simulink model "bai2111"  (R2022b)
settings: Solver=VariableStepAuto  StartTime=0.0  StopTime=20  RelTol=1e-8
values from neighbouring files (symbols this model uses):
  k0 = -8    [bai21111.m]
  k1 = -1    [bai21111.m]
  T = T_list(k)    [bai21111.m]
settings Model: Creator=admin  LastModifiedBy=admin

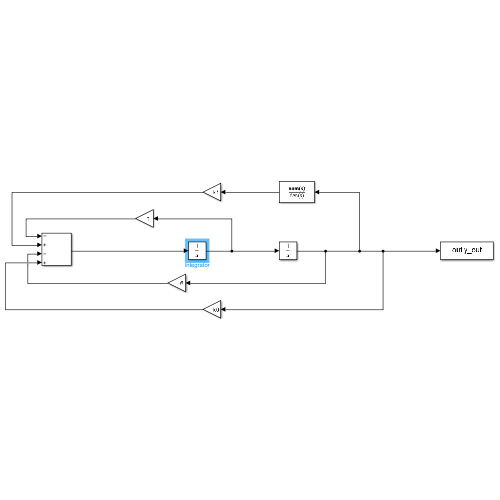
[thumbnail: Simulink's stored preview of the top-level diagram]
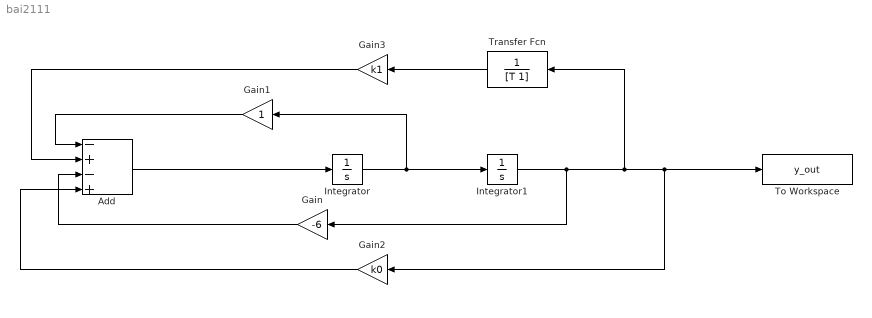
== system bai2111 ==
  Add : Sum  Inputs=-+-+
  Gain : Gain  Gain=-6
  Gain1 : Gain
  Gain2 : Gain  Gain=k0
  Gain3 : Gain  Gain=k1
  Integrator : Integrator  InitialCondition=5
  Integrator1 : Integrator
  To Workspace : ToWorkspace  VariableName=y_out  SaveFormat=Structure With Time  SampleTime=-1
  Transfer Fcn : TransferFcn  Denominator=[T 1]
  wires:
  Gain2/1 -> Add/4
  Integrator/1 -> Gain1/1, Integrator1/1
  Integrator1/1 -> Gain/1, Gain2/1, To Workspace/1, Transfer Fcn/1
  Gain3/1 -> Add/2
  Gain/1 -> Add/3
  Transfer Fcn/1 -> Gain3/1
  Gain1/1 -> Add/1
  Add/1 -> Integrator/1
